simulink model "sampleModel1445_1_sub"  (R2023a)
settings: Solver=VariableStepAuto  StartTime=0.0  StopTime=10.0  RelTol=1e-3
libraries: hdlsllib x5, simulink x2
settings Model: Creator=user1  LastModifiedBy=user1
settings OptimizationCC: BlockReduction=off  ConditionallyExecuteInputs=off

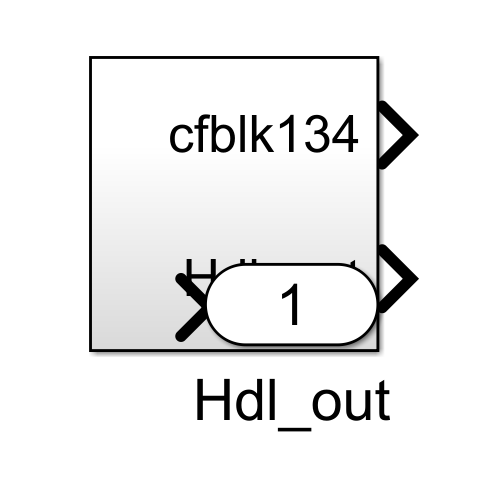
[thumbnail: Simulink's stored preview of the top-level diagram]
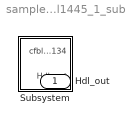
== system sampleModel1445_1_sub ==
  Subsystem : Subsystem
  Hdl_out : Outport  OutDataTypeStr=uint8

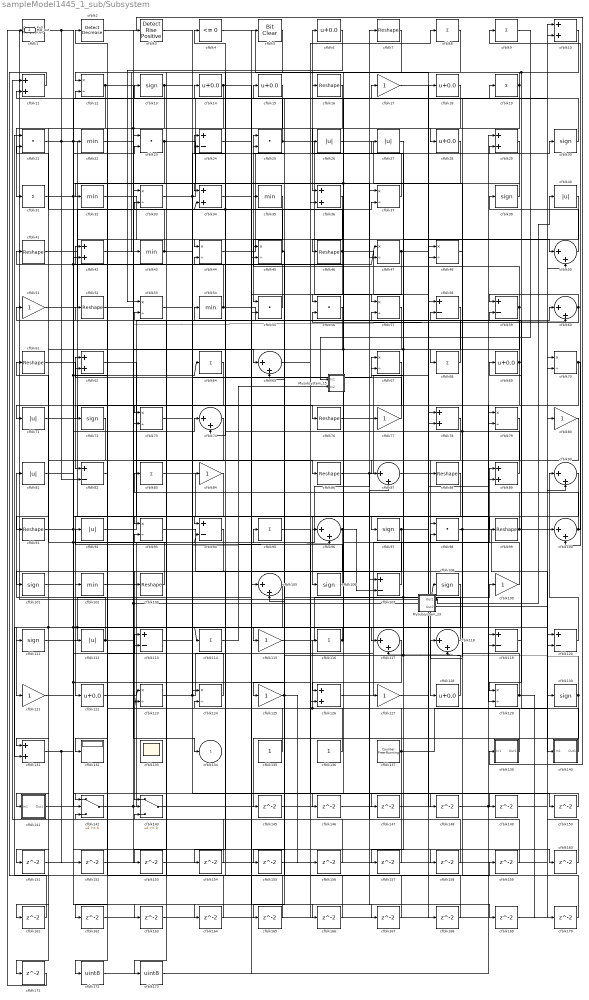
== system sampleModel1445_1_sub/Subsystem ==
  Mysubsystem_15 : Subsystem  TreatAsAtomicUnit=on  RTWFcnName=Mysubsystem_15
      settings: RTWFcnNameOpts=User specified  RTWFileNameOpts=Use function name
  Mysubsystem_23 : Subsystem  TreatAsAtomicUnit=on  RTWFcnName=Mysubsystem_23
      settings: RTWFcnNameOpts=User specified  RTWFileNameOpts=Use function name
  cfblk1 : hdlsllib/Logic and Bit Operations/Detect Fall Nonpositive  vinit=0  OutDataTypeStr=uint8
  cfblk{10..11,29,34,36,42,62,78,89,126,131} (11 alike) : Sum  OutDataTypeStr=uint8
  cfblk{50,60,65,74,87,90,96,100,105,117..118} (11 alike) : Sum  Inputs=|++  OutDataTypeStr=uint8
  cfblk{13,30,39,72,97,101,106,108,111,130} (10 alike) : Signum
  cfblk{22,32,35,43,54,102} (6 alike) : MinMax  OutDataTypeStr=uint8
  cfblk{7,16,41,46,52,61,76,86,88,91,99,103} (12 alike) : Reshape
  cfblk{24,58..59,82,94,107,113,119..120} (9 alike) : Sum  Inputs=+-  OutDataTypeStr=uint8
  cfblk{17,51,77,80,84,109,115,121,125,127} (10 alike) : Gain  OutDataTypeStr=uint8
  cfblk{26..27,40,71,81,92,112} (7 alike) : Abs  OutDataTypeStr=uint8  SaturateOnIntegerOverflow=off
  cfblk{8..9,19,31,64,68,83,95,114,116} (10 alike) : Sum  Inputs=+  OutDataTypeStr=uint8
  cfblk{12,33,37,44..45,47..48,53,57,67,70,73,79,93,123..124,129} (17 alike) : Product  Inputs=*/  OutDataTypeStr=uint8  RndMeth=Zero  SaturateOnIntegerOverflow=on
  cfblk{6,14..15,18,28,69,122,128} (8 alike) : Bias  Bias=0.0  SaturateOnIntegerOverflow=off
  cfblk132 : Display
  cfblk133 : Scope
      settings: Floating=on
  cfblk135 : Constant  OutDataTypeStr=uint8  SampleTime=-1
  cfblk136 : Constant  OutDataTypeStr=uint8  SampleTime=-1
  cfblk137 : hdlsllib/Sources/Counter Free-Running  NumBits=16  tsamp=-1
  cfblk139 : Subsystem
      settings: LibrarySourceBlock=|
      | hdlsllib/Ports &
      | Subsystems/Subsystem
  cfblk140 : Subsystem
      settings: LibrarySourceBlock=|
      | hdlsllib/Ports &
      | Subsystems/Subsystem
  cfblk141 : Subsystem
      settings: LibrarySourceBlock=|
      | hdlsllib/Ports &
      | Subsystems/Subsystem
  cfblk142 : Switch  OutDataTypeStr=uint8  SaturateOnIntegerOverflow=off  InputSameDT=off
  cfblk143 : Switch  OutDataTypeStr=uint8  SaturateOnIntegerOverflow=off  InputSameDT=off
  cfblk{145..171} (27 alike) : Delay  SampleTime=1
  cfblk172 : DataTypeConversion  OutDataTypeStr=uint8  SaturateOnIntegerOverflow=off  RndMeth=Floor
  cfblk173 : DataTypeConversion  OutDataTypeStr=uint8  SaturateOnIntegerOverflow=off  RndMeth=Floor
  cfblk2 : simulink/Logic and Bit Operations/Detect Decrease  vinit=0.0  OutDataTypeStr=uint8
      settings: LibrarySourceBlock=|
      | hdlsllib/Logic and Bit
      | Operations/Detect
      | Decrease
  cfblk{21,23,25,55..56,98} (6 alike) : DotProduct  OutDataTypeStr=uint8
  cfblk3 : hdlsllib/Logic and Bit Operations/Detect Rise Positive  vinit=0  OutDataTypeStr=uint8
  cfblk4 : hdlsllib/Logic and Bit Operations/Compare To Zero  relop=<=  OutDataTypeStr=uint8
  cfblk5 : simulink/Logic and Bit Operations/Bit Clear  iBit=0
      settings: LibrarySourceBlock=|
      | hdlsllib/Logic and Bit
      | Operations/Bit Clear
  cfblk134 : Outport  OutDataTypeStr=uint8  VectorParamsAs1DForOutWhenUnconnected=off
  Hdl_out : Outport  Port=2  OutDataTypeStr=uint8
  wires:
  cfblk108/1 -> cfblk151/1, cfblk131/2
  cfblk112/1 -> cfblk134/1, cfblk81/1
  cfblk88/1 -> cfblk122/1
  cfblk94/1 -> cfblk142/1
  cfblk7/1 -> cfblk43/1
  cfblk26/1 -> cfblk68/1
  cfblk111/1 -> cfblk45/2, cfblk114/1
  cfblk115/1 -> cfblk109/1
  cfblk6/1 -> cfblk53/1
  cfblk80/1 -> cfblk101/1
  cfblk21/1 -> cfblk82/2, cfblk163/1, cfblk97/1
  cfblk139/1(Out1) -> cfblk123/1, cfblk116/1
  cfblk41/1 -> cfblk50/1
  cfblk137/1 -> cfblk90/2, cfblk42/1, cfblk11/1
  cfblk113/1 -> cfblk67/1
  cfblk32/1 -> cfblk44/1
  cfblk128/1 -> cfblk25/2, cfblk27/1
  cfblk142/1 -> cfblk95/1, cfblk60/2, cfblk108/1
  cfblk92/1 -> cfblk7/1
  cfblk105/1 -> cfblk121/1
  cfblk87/1 -> cfblk48/1
  cfblk143/1 -> cfblk80/1, cfblk79/1
  cfblk61/1 -> cfblk82/1
  cfblk23/1 -> cfblk47/2, cfblk102/1
  cfblk100/1 -> cfblk4/1, cfblk9/1
  cfblk103/1 -> cfblk61/1
  cfblk57/1 -> cfblk96/1, cfblk131/1
  cfblk84/1 -> cfblk93/1
  cfblk37/1 -> cfblk6/1
  cfblk28/1 -> cfblk123/2, cfblk126/1
  cfblk45/1 -> cfblk21/2, cfblk125/1
  cfblk62/1 -> cfblk105/1
  cfblk126/1 -> cfblk58/1
  cfblk25/1 -> cfblk12/2, cfblk57/1
  cfblk60/1 -> cfblk56/2, cfblk59/1
  cfblk69/1 -> cfblk129/2, cfblk54/1
  cfblk86/1 -> cfblk169/1, cfblk18/1
  cfblk50/1 -> cfblk39/1
  cfblk136/1 -> cfblk15/1
  cfblk2/1 -> cfblk139/1(In1)
  cfblk119/1 -> cfblk69/1
  cfblk35/1 -> cfblk55/1
  cfblk96/1 -> cfblk154/1, cfblk107/2
  cfblk74/1 -> cfblk132/1
  cfblk43/1 -> cfblk147/1, cfblk33/2
  cfblk65/1 -> cfblk8/1
  cfblk27/1 -> cfblk87/1
  cfblk106/1 -> cfblk92/1
  cfblk78/1 -> cfblk128/1
  cfblk58/1 -> cfblk157/1, cfblk112/1
  cfblk36/1 -> cfblk46/1
  cfblk109/1 -> cfblk51/1
  cfblk129/1 -> cfblk170/1, cfblk14/1
  cfblk127/1 -> cfblk19/1
  cfblk19/1 -> cfblk28/1, cfblk12/1
  cfblk54/1 -> cfblk60/1, cfblk2/1
  cfblk101/1 -> cfblk64/1, cfblk17/1, cfblk47/1
  cfblk12/1 -> cfblk65/1, cfblk31/1
  cfblk140/1(Out1) -> cfblk59/2
  cfblk64/1 -> cfblk141/1(In1)
  cfblk42/1 -> cfblk86/1
  cfblk123/1 -> cfblk26/1, cfblk89/1
  cfblk46/1 -> cfblk65/2, cfblk24/2, cfblk88/1
  cfblk130/1 -> cfblk145/1, cfblk117/2
  cfblk48/1 -> cfblk98/1
  cfblk97/1 -> cfblk161/1, cfblk89/2
  cfblk53/1 -> cfblk120/2
  cfblk44/1 -> cfblk30/1
  cfblk79/1 -> cfblk91/1
  cfblk120/1 -> cfblk90/1
  cfblk98/1 -> cfblk118/2, cfblk130/1
  cfblk99/1 -> cfblk83/1, cfblk70/1
  cfblk59/1 -> cfblk111/1, cfblk25/1
  cfblk39/1 -> cfblk32/1
  cfblk3/1 -> cfblk124/1
  cfblk22/1 -> cfblk3/1
  cfblk102/1 -> cfblk143/1
  cfblk71/1 -> cfblk76/1
  cfblk93/1 -> cfblk119/2
  cfblk16/1 -> cfblk71/1
  cfblk125/1 -> cfblk156/1, cfblk155/1
  cfblk107/1 -> cfblk45/1
  cfblk30/1 -> cfblk13/1
  cfblk52/1 -> cfblk35/1
  cfblk10/1 -> cfblk74/2, cfblk129/1
  cfblk91/1 -> cfblk94/1, cfblk166/1, cfblk126/2
  cfblk121/1 -> cfblk94/2, cfblk23/2
  cfblk18/1 -> cfblk36/1
  cfblk122/1 -> cfblk77/1
  cfblk1/1 -> cfblk22/1, cfblk99/1
  cfblk77/1 -> cfblk62/1
  cfblk29/1 -> cfblk103/1
  cfblk15/1 -> cfblk73/1
  cfblk83/1 -> cfblk127/1
  cfblk118/1 -> cfblk67/2, cfblk41/1
  cfblk89/1 -> cfblk58/2, cfblk34/2, cfblk11/2
  cfblk90/1 -> cfblk106/1
  cfblk47/1 -> cfblk55/2, cfblk29/2
  cfblk68/1 -> cfblk57/2
  cfblk33/1 -> cfblk96/2, cfblk10/1
  cfblk55/1 -> cfblk24/1
  cfblk131/1 -> cfblk152/1, cfblk113/1
  cfblk40/1 -> cfblk117/1
  cfblk4/1 -> cfblk78/1
  cfblk76/1 -> cfblk37/1
  cfblk31/1 -> cfblk34/1, cfblk164/1, cfblk113/2
  cfblk14/1 -> cfblk149/1, cfblk42/2, cfblk73/2
  cfblk116/1 -> cfblk115/1, cfblk16/1
  cfblk13/1 -> cfblk172/1, cfblk84/1
  cfblk70/1 -> cfblk72/1, cfblk100/2
  cfblk51/1 -> cfblk37/2
  cfblk135/1 -> cfblk124/2
  cfblk124/1 -> cfblk52/1
  cfblk141/1(Out1) -> cfblk74/1
  cfblk8/1 -> cfblk56/1
  cfblk145/1 -> cfblk87/2
  cfblk117/1 -> cfblk146/1
  cfblk146/1 -> cfblk78/2
  cfblk147/1 -> cfblk48/2
  cfblk73/1 -> cfblk148/1
  cfblk148/1 -> cfblk100/1
  cfblk149/1 -> cfblk70/2
  cfblk95/1 -> cfblk150/1
  cfblk150/1 -> cfblk142/2
  cfblk151/1 -> cfblk23/1
  cfblk152/1 -> cfblk10/2
  cfblk67/1 -> cfblk153/1
  cfblk153/1 -> cfblk93/2
  cfblk154/1 -> cfblk33/1
  cfblk155/1 -> cfblk79/2
  cfblk156/1 -> cfblk143/2
  cfblk157/1 -> cfblk142/3
  cfblk81/1 -> cfblk158/1
  cfblk158/1 -> cfblk107/1
  cfblk11/1 -> cfblk159/1
  cfblk159/1 -> cfblk98/2
  cfblk34/1 -> cfblk160/1
  cfblk160/1 -> cfblk120/1
  cfblk161/1 -> cfblk21/1
  cfblk82/1 -> cfblk162/1
  cfblk162/1 -> cfblk119/1
  cfblk163/1 -> cfblk36/2
  cfblk164/1 -> cfblk143/3
  cfblk56/1 -> cfblk165/1
  cfblk165/1 -> cfblk44/2
  cfblk166/1 -> cfblk62/2
  cfblk24/1 -> cfblk167/1
  cfblk167/1 -> cfblk105/2
  cfblk17/1 -> cfblk168/1
  cfblk168/1 -> cfblk53/2
  cfblk169/1 -> cfblk50/2
  cfblk170/1 -> cfblk118/1
  cfblk72/1 -> cfblk171/1
  cfblk171/1 -> cfblk1/1
  cfblk172/1 -> cfblk5/1
  cfblk5/1 -> cfblk173/1
  cfblk173/1 -> cfblk29/1
  cfblk9/1 -> Mysubsystem_15/1(In1)
  cfblk114/1 -> Mysubsystem_15/2(In2)
  Mysubsystem_23/1(Out1) -> Hdl_out/1, cfblk40/1
  Mysubsystem_23/2(Out2) -> cfblk140/1(In1)

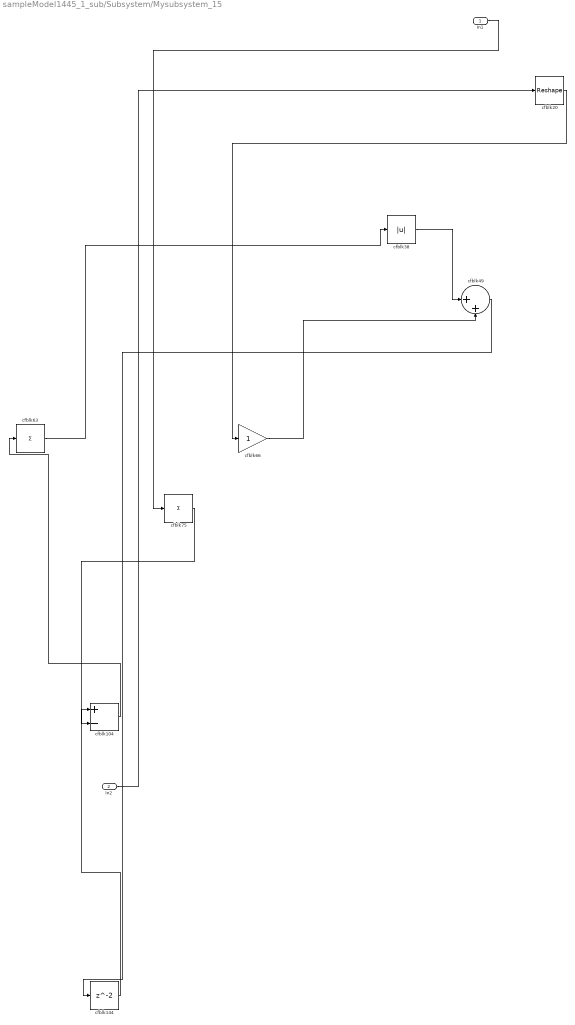
== system sampleModel1445_1_sub/Subsystem/Mysubsystem_15 ==
  In1 : Inport
  In2 : Inport  Port=2
  cfblk104 : Sum  Inputs=+-
  cfblk144 : Delay  SampleTime=1
  cfblk20 : Reshape
  cfblk38 : Abs  SaturateOnIntegerOverflow=off
  cfblk49 : Sum  Inputs=|++
  cfblk63 : Sum  Inputs=+
  cfblk66 : Gain
  cfblk75 : Sum  Inputs=+
  wires:
  In2/1 -> cfblk20/1
  In1/1 -> cfblk75/1
  cfblk144/1 -> cfblk104/1
  cfblk20/1 -> cfblk66/1
  cfblk75/1 -> cfblk104/2
  cfblk66/1 -> cfblk49/2
  cfblk38/1 -> cfblk49/1
  cfblk49/1 -> cfblk144/1
  cfblk63/1 -> cfblk38/1
  cfblk104/1 -> cfblk63/1

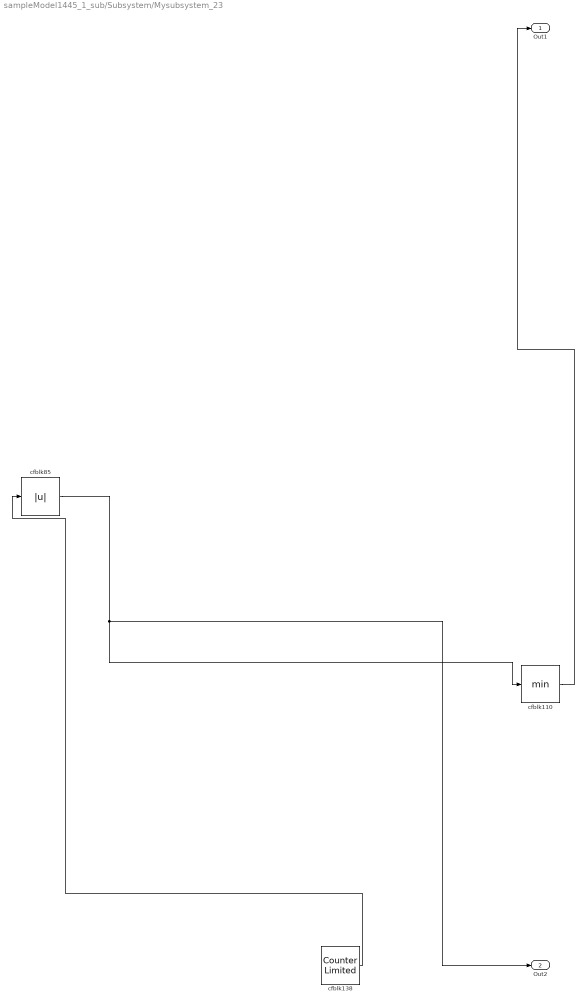
== system sampleModel1445_1_sub/Subsystem/Mysubsystem_23 ==
  cfblk110 : MinMax
  cfblk138 : hdlsllib/Sources/Counter Limited  uplimit=7  tsamp=-1
  cfblk85 : Abs  SaturateOnIntegerOverflow=off
  Out1 : Outport
  Out2 : Outport  Port=2
  wires:
  cfblk110/1 -> Out1/1
  cfblk85/1 -> cfblk110/1, Out2/1
  cfblk138/1 -> cfblk85/1

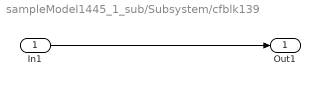
== system sampleModel1445_1_sub/Subsystem/cfblk139 ==
  In1 : Inport
  Out1 : Outport
  wires:
  In1/1 -> Out1/1

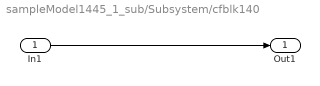
== system sampleModel1445_1_sub/Subsystem/cfblk140 ==
  In1 : Inport
  Out1 : Outport
  wires:
  In1/1 -> Out1/1

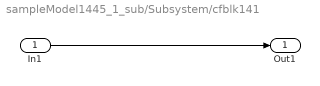
== system sampleModel1445_1_sub/Subsystem/cfblk141 ==
  In1 : Inport
  Out1 : Outport
  wires:
  In1/1 -> Out1/1
